simulink model "prob2_week1"  (R2020b)
settings: Solver=VariableStepAuto  StartTime=0.0  StopTime=10.0  RelTol=1e-3
undefined symbols (not defined in the file): b, k1, k2, m1, m2
settings Model: Creator=Pulkit Khandelwal  LastModifiedBy=Pulkit Khandelwal

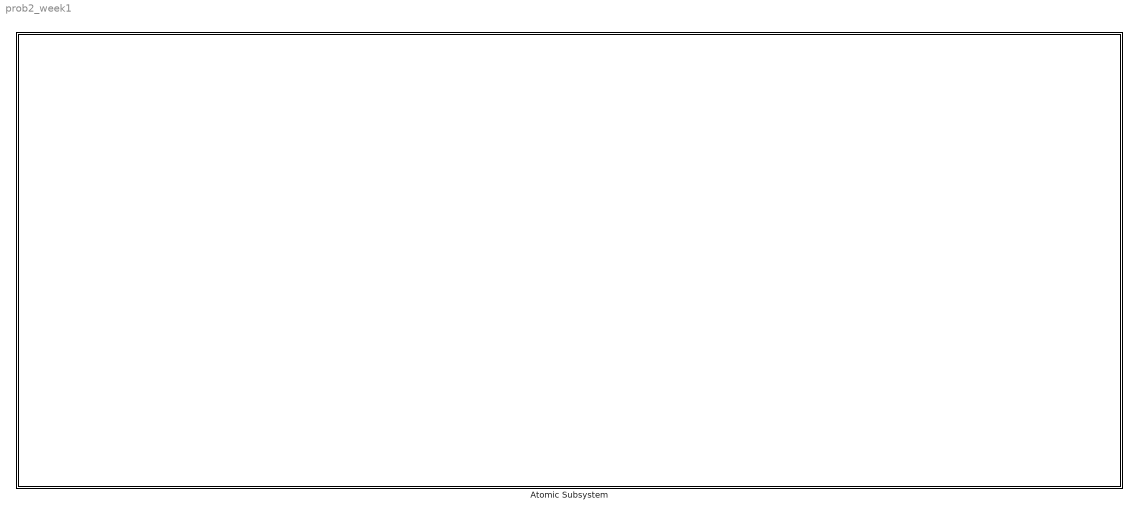
== system prob2_week1 ==
  Atomic Subsystem : Subsystem  TreatAsAtomicUnit=on

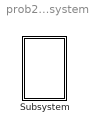
== system prob2_week1/Atomic Subsystem ==
  Subsystem : Subsystem  TreatAsAtomicUnit=on

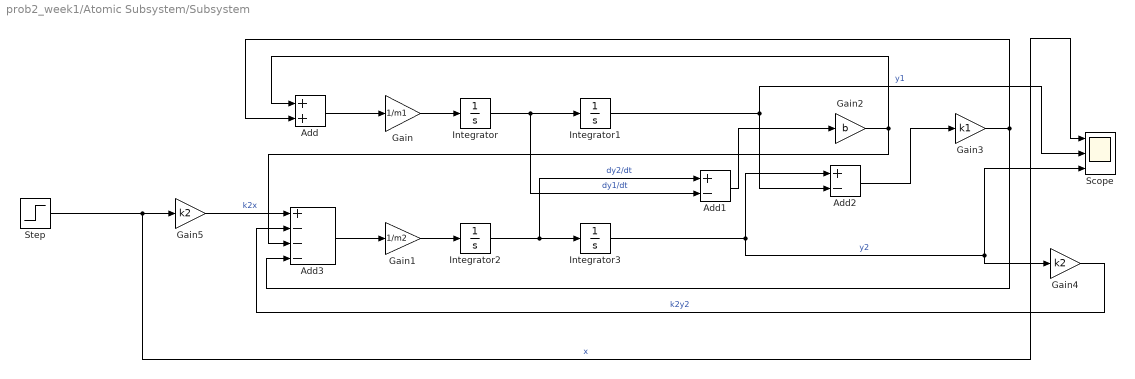
== system prob2_week1/Atomic Subsystem/Subsystem ==
  Add : Sum
  Add1 : Sum  Inputs=+-
  Add2 : Sum  Inputs=+-
  Add3 : Sum  Inputs=+---
  Gain : Gain  Gain=1/m1
  Gain1 : Gain  Gain=1/m2
  Gain2 : Gain  Gain=b
  Gain3 : Gain  Gain=k1
  Gain4 : Gain  Gain=k2
  Gain5 : Gain  Gain=k2
  Integrator{,1..3} (4 alike) : Integrator
  Scope : Scope  NumInputPorts=3
  Step : Step  Time=5  SampleTime=0
  wires:
  Add3/1 -> Gain1/1
  Gain3/1 -> Add/2, Add3/4
  Gain1/1 -> Integrator2/1
  Integrator1/1 -> Add2/2, Scope/2  "y1"
  Step/1 -> Scope/1, Gain5/1  "x"
  Gain5/1 -> Add3/1  "k2x"
  Gain2/1 -> Add3/3, Add/1
  Gain4/1 -> Add3/2  "k2y2"
  Integrator2/1 -> Add1/1, Integrator3/1  "dy2/dt"
  Integrator/1 -> Add1/2, Integrator1/1  "dy1/dt"
  Integrator3/1 -> Scope/3, Gain4/1, Add2/1  "y2"
  Gain/1 -> Integrator/1
  Add/1 -> Gain/1
  Add1/1 -> Gain2/1
  Add2/1 -> Gain3/1
